simulink model "CO2_Electrolyzer"  (R2025a)
settings: Solver=VariableStepAuto  StartTime=0.0  StopTime=3600  RelTol=1e-3
PreLoadFcn:
  | run('params_co2el.m');
StartFcn:
  | run(fullfile(fileparts(bdroot),'params_co2el.m'));
values from neighbouring files (symbols this model uses):
  A_cm2 = 200    [params_co2el.m]
  F = 96485.33212    [params_co2el.m]
  j_tab_mAcm2 = [0 ... (first row only)    [params_co2el.m]
  MW_CO = 28.0101e-3    (= 0.0280101)    [params_co2el.m]
  MW_CO2 = 44.0095e-3    (= 0.0440095)    [params_co2el.m]
  MW_H2 = 2.01588e-3    (= 0.00201588)    [params_co2el.m]
  N_cell = 200    [params_co2el.m]
  p_bp = [0 ... (first row only)    [params_co2el.m]
  P_stack_max_W = p_max * (N_cell*A_cm2) / 1000    [params_co2el.m]
  V_tab = [0 ... (first row only)    [params_co2el.m]
libraries: simulink x1
settings Model: Creator=ALW  LastModifiedBy=ALW

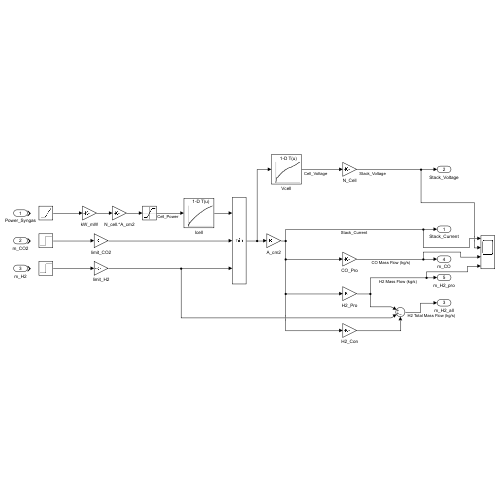
[thumbnail: Simulink's stored preview of the top-level diagram]
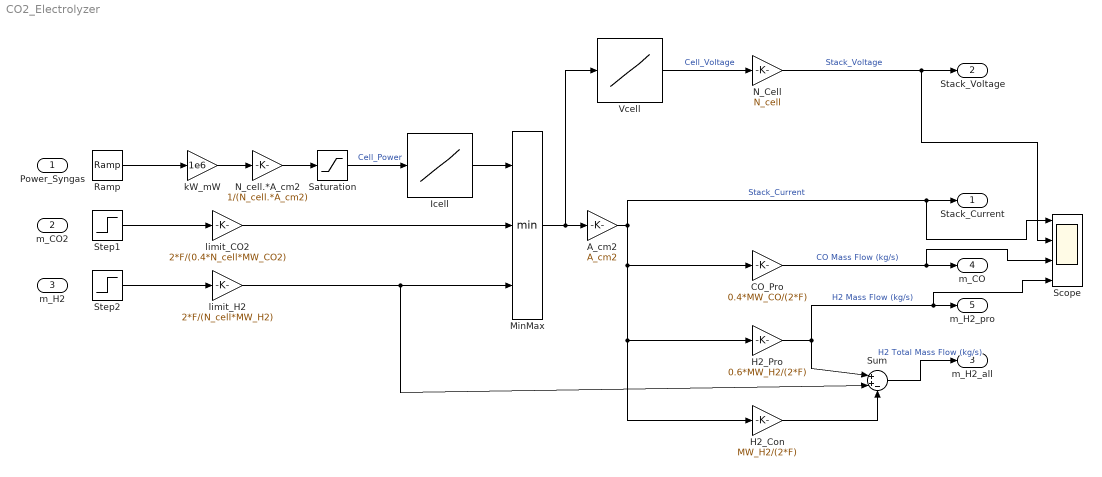
== system CO2_Electrolyzer ==
  Power_Syngas : Inport
  m_CO2 : Inport  Port=2
  m_H2 : Inport  Port=3
  A_cm2 : Gain  Gain=A_cm2
  CO_Pro : Gain  Gain=0.4*MW_CO/(2*F)
  H2_Con : Gain  Gain=MW_H2/(2*F)
  H2_Pro : Gain  Gain=0.6*MW_H2/(2*F)
  Icell : Lookup_n-D  NumberOfTableDimensions=1  BreakpointsForDimension1=p_bp  Table=j_tab_mAcm2  InternalRulePriority=Speed  RndMeth=Simplest
  MinMax : MinMax  Inputs=3
  N_Cell : Gain  Gain=N_cell
  N_cell.*A_cm2 : Gain  Gain=1/(N_cell.*A_cm2)
  Ramp : simulink/Sources/Ramp  slope=1  start=0  InitialOutput=0
  Saturation : Saturate  UpperLimit=P_stack_max_W  LowerLimit=0
  Scope : Scope  NumInputPorts=4
      settings: ActiveDisplayString=4  ActiveDisplayYMinimum=-0.00046042184065135877  ActiveDisplayYMaximum=0.00414379656586223
  Step1 : Step  After=0.5  SampleTime=0
  Step2 : Step  After=0.5  SampleTime=0
  Sum : Sum  Inputs=|++-
  Vcell : Lookup_n-D  NumberOfTableDimensions=1  BreakpointsForDimension1=j_tab_mAcm2  Table=V_tab  InternalRulePriority=Speed  RndMeth=Simplest
  kW_mW : Gain  Gain=1e6
  limit_CO2 : Gain  Gain=2*F/(0.4*N_cell*MW_CO2)
  limit_H2 : Gain  Gain=2*F/(N_cell*MW_H2)
  Stack_Current : Outport
  Stack_Voltage : Outport  Port=2
  m_H2_all : Outport  Port=3
  m_CO : Outport  Port=4
  m_H2_pro : Outport  Port=5
  wires:
  Ramp/1 -> kW_mW/1
  kW_mW/1 -> N_cell.*A_cm2/1
  N_cell.*A_cm2/1 -> Saturation/1
  Saturation/1 -> Icell/1  "Cell_Power"
  Icell/1 -> MinMax/1
  A_cm2/1 -> CO_Pro/1, H2_Con/1, H2_Pro/1, Scope/1, Stack_Current/1  "Stack_Current"
  Step1/1 -> limit_CO2/1
  Step2/1 -> limit_H2/1
  limit_H2/1 -> Sum/2, MinMax/3
  limit_CO2/1 -> MinMax/2
  MinMax/1 -> Vcell/1, A_cm2/1
  Vcell/1 -> N_Cell/1  "Cell_Voltage"
  N_Cell/1 -> Scope/2, Stack_Voltage/1  "Stack_Voltage"
  H2_Pro/1 -> Sum/1, Scope/4, m_H2_pro/1  "H2 Mass Flow (kg/s)"
  H2_Con/1 -> Sum/3
  Sum/1 -> m_H2_all/1  "H2 Total Mass Flow (kg/s)"
  CO_Pro/1 -> Scope/3, m_CO/1  "CO Mass Flow (kg/s)"
